simulink model "mpc2dof_lat_lon"  (R2022a)
settings: Solver=VariableStepAuto  StartTime=0.0  StopTime=5  RelTol=1e-3
PreLoadFcn:
  | preload
values from neighbouring files (symbols this model uses):
  aubr = [-8 -7.95 -7.9 -7.85 -7.8 -7.75 -7.7 -7.65 -7.6 -7.55 -7.5 -7.45 ... (261 elements, 1x261)]    [biaodingbiao.mat]
  tablebr = [-5.15763257253 -5.44224077841 -5.70856006024 -6.19075802128 -6.74229369367 -6.72484954572 -6.64837028644 -6.64755997194 -6.64688047281 -6.64617751235 -6.6454745519 -6.76173851825 ... (261261 elements, 1001x261)]    [biaodingbiao.mat]
  vubr = [0 0.05 0.1 0.15 0.2 0.25 0.3 0.35 0.4 0.45 0.5 0.55 ... (1001 elements, 1x1001)]    [biaodingbiao.mat]
libraries: slpidlib x3, Solver_SF x1
settings Model: Creator=化  LastModifiedBy=化

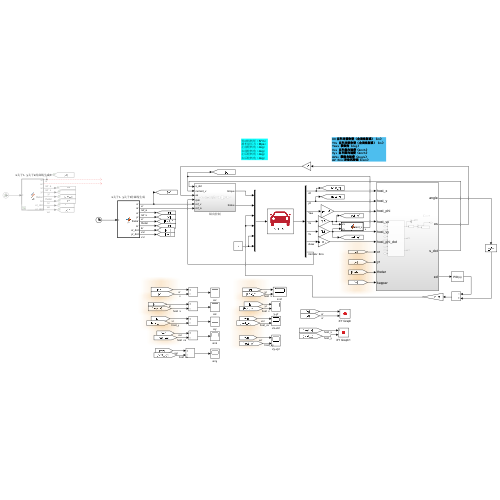
[thumbnail: Simulink's stored preview of the top-level diagram]
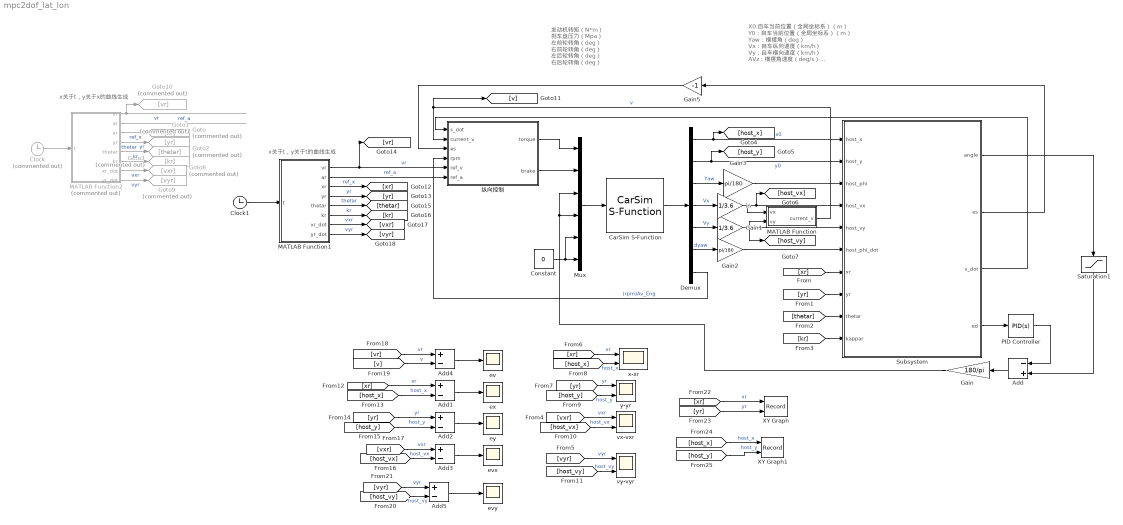
== system mpc2dof_lat_lon ==
  note: 发动机转矩（N*m）
      | 刹车盘压力（Mpa）
      | 左前轮转角（deg）
      | 右前轮转角（deg）
      | 左后轮转角（deg）
      | 右后轮转角（deg）
  note: X0:自车当前位置（全局坐标系）（m）
      | Y0：自车当前位置（全局坐标系）（m）
      | Yaw：横摆角（deg）
      | Vx：自车纵向速度（km/h）
      | Vy：自车横向速度（km/h）
      | AVz：横摆角速度（deg/s）
      | AV_Eng:发动机转速（rpm）
  note: x关于t，y关于x的曲线生成
  note: x关于t，y关于t的曲线生成
  Add : Sum  Inputs=-+
  Add{1..5} (5 alike) : Sum  Inputs=+-
  CarSim S-Function : Solver_SF/CarSim S-Function  Priority=1  SIMFILE=simfile.sim  Run_RTs=off  vs_state_ind=Run  StopMode_ind=Vehicle Model
  Clock : Clock  Commented=on
  Clock1 : Clock
  Constant : Constant  Value=0
  Demux : Demux  Outputs=7
  Gain : Gain  Gain=180/pi
  Gain1 : Gain  Gain=1/3.6
  Gain2 : Gain  Gain=pi/180
  Gain3 : Gain  Gain=pi/180
  Gain5 : Gain  Gain=-1
  Goto : Goto  Commented=on  GotoTag=xr
  Goto1 : Goto  Commented=on  GotoTag=yr
  Goto10 : Goto  Commented=on  GotoTag=vr
  Goto2 : Goto  Commented=on  GotoTag=thetar
  Goto3 : Goto  Commented=on  GotoTag=kr
  Goto8 : Goto  Commented=on  GotoTag=vxr
  Goto9 : Goto  Commented=on  GotoTag=vyr
  MATLAB Function : MATLAB Function  TreatAsAtomicUnit=on
  MATLAB Function1 : MATLAB Function  TreatAsAtomicUnit=on
  MATLAB Function2 : MATLAB Function  Commented=on  TreatAsAtomicUnit=on
  Mux : Mux  Inputs=6
  PID Controller : slpidlib/PID Controller  Controller=PID  Form=Parallel  TimeDomain=Continuous-time  UseExternalTs=off  SampleTime=-1  IntegratorMethod=Forward Euler  FilterMethod=Forward Euler  ControllerParametersSource=internal  P=0  I=3  UseKiTs=off  D=0  N=100  UseFilter=on  TunerSelectOption=Transfer Function Based (PID Tuner App)  InitialConditionSource=internal  InitialConditionForIntegrator=0  InitialConditionForFilter=0  DifferentiatorICPrevScaledInput=0  ExternalReset=none  TrackingMode=off  Kt=1  LimitOutput=off  SatLimitsSource=internal  UpperSaturationLimit=inf  LowerSaturationLimit=-inf  LinearizeAsGain=on  AntiWindupMode=none  Kb=1  POutMin=[]  POutMax=[]  IOutMin=[]  IOutMax=[]  DOutMin=[]  DOutMax=[]  NOutMin=[]  NOutMax=[]  SumOutMin=[]  SumOutMax=[]  SaturationOutMin=[]  SaturationOutMax=[]  PParamMin=[]  PParamMax=[]  IParamMin=[]  IParamMax=[]  DParamMin=[]  DParamMax=[]  NParamMin=[]  NParamMax=[]  KbParamMin=[]  KbParamMax=[]  KtParamMin=[]  KtParamMax=[]  KbOutMin=[]  KbOutMax=[]  KtOutMin=[]  KtOutMax=[]  IntegratorOutMin=[]  IntegratorOutMax=[]  FilterOutMin=[]  FilterOutMax=[]  SumI1OutMin=[]  SumI1OutMax=[]  SumI2OutMin=[]  SumI2OutMax=[]  SumI3OutMin=[]  SumI3OutMax=[]  SumI4OutMin=[]  SumI4OutMax=[]  SumDOutMin=[]  SumDOutMax=[]  DifferentiatorOutMin=[]  DifferentiatorOutMax=[]  FilterDiffOutCoefMin=[]  FilterDiffOutCoefMax=[]  ReciprocalOutMin=[]  ReciprocalOutMax=[]  SumDenOutMin=[]  SumDenOutMax=[]  SumNumOutMin=[]  SumNumOutMax=[]  DivideOutMin=[]  DivideOutMax=[]  UdiffTsProdOutMin=[]  UdiffTsProdOutMax=[]  NTsProdOutMin=[]  NTsProdOutMax=[]  UintegralTsProdOutMin=[]  UintegralTsProdOutMax=[]  UngainTsProdOutMin=[]  UngainTsProdOutMax=[]  IntegratorContinuousStateAttributes=''  IntegratorStateMustResolveToSignalObject=off  IntegratorRTWStateStorageClass=Auto  FilterContinuousStateAttributes=''  FilterStateMustResolveToSignalObject=off  FilterRTWStateStorageClass=Auto  ParallelPVariant=InternalParameters  IdealPVariant=Disabled  IVariant=InternalParameters  DVariant=InternalParameters  IntegratorVariant=Continuous  SatVariant=Disabled  AWVariant=Passthrough  PCopyVariant=Disabled  TRVariant=Disabled  FdbkBlocksVariant=Forward  IdealPFdbkVariant=Disabled  SatFdbkVariant=Disabled  DerivativeFilterVariant=ContFilter  NVariant=InternalParameters  NCopyVariant=Disabled  FilterICVariant=InternalICsFilter  IntegratorICVariant=InternalICs  ExternalResetVariant=Disabled  TRSumVariant=Passthrough  SumFdbkVariant=Disabled  SumVariant=Sum_PID  TsampFilterVariant=InternalTs  TsampNgainVariant=Passthrough  TsampIntegralVariant=Passthrough  ExternalSaturationOutDataTypeStr=Inherit: Same as second input  aMode=0
  Saturation1 : Saturate  UpperLimit=1  LowerLimit=-1
  Subsystem : Subsystem
  XY Graph : Record  FileSettingsInternal="{\"entries\":[{\"content\":{\"excelSettings\":{\"content\":{},\"type\":\"Streamout.ExcelSettings\"}},\"type\":\"Streamout.FileSettingStorage\",\"uuid\":\"0858db11-d2cd-44ce-b257-d2a84fc32b74\"}],\"packageUris\":[\"http://schema.mathworks.com/mf0/streamout_blocks/R2020a\"],\"version\":\"1.0\"}"  Layout=[1 1]  SignalsInternal="{\"entries\":[{\"content\":{\"signals\":[{\"content\":{\"blockPath\":[\"mpc2dof_lat_lon/XY Graph\"],\"channel\":[],\"dimensions\":[1],\"domain\":\"mpc2dof_lat_lon/XY Graph\",\"lineColor\":\"#a2142f\",\"plots\":[1],\"port\":1,\"sid\":[\"\"],\"signalID\":657,\"signalName\":\"xr\"},\"type\":\"RecordBlkView.Signal\",\"uuid\":\"f73990f6-9684-49e6-9729-589b4f1455ea\"},{\"content\":{\"blockPath\":[\"mpc2dof_lat_lon/XY Graph\"],\"channel\":[],\"dimensions\":[1],\"domain\":\"mpc2dof_lat_lon/XY Graph\",\"lineColor\":\"#139fff\",\"plots\":[1],\"port\":2,\"sid\":[\"\"],\"signalID\":661,\"signalName\":\"yr\"},\"type\":\"RecordBlkView.Signal\",\"uuid\":\"39c842ae-e1c5-41be-97e8-3fe2b4711ec7\"}]},\"type\":\"RecordBlkView.InputSignals\",\"uuid\":\"8e38f882-027b-4b6b-b800-43f1a68d75de\"}],\"packageUris\":[\"http://schema.mathworks.com/mf0/streamout_blocks/R2020a\"],\"version\":\"1.0\"}"  VisualizationBindings="{\"xyplotplugin\":{\"info\":[{\"series\":[{\"bindingParametersList\":[{\"parameter\":\"X-Axis\",\"signalID\":657,\"signalName\":\"xr\"},{\"parameter\":\"Y-Axis\",\"signalID\":661,\"signalName\":\"yr\"}],\"seriesID\":62107}],\"subplotID\":1}]}}"  CompatibilityTag=XY
  XY Graph1 : Record  FileSettingsInternal="{\"entries\":[{\"content\":{\"excelSettings\":{\"content\":{},\"type\":\"Streamout.ExcelSettings\"}},\"type\":\"Streamout.FileSettingStorage\",\"uuid\":\"ff16b887-db1a-418b-9102-38758cb726a0\"}],\"packageUris\":[\"http://schema.mathworks.com/mf0/streamout_blocks/R2020a\"],\"version\":\"1.0\"}"  Layout=[1 1]  SignalsInternal="{\"entries\":[{\"content\":{\"signals\":[{\"content\":{\"blockPath\":[\"mpc2dof_lat_lon/XY Graph1\"],\"channel\":[],\"dimensions\":[1],\"domain\":\"mpc2dof_lat_lon/XY Graph1\",\"lineColor\":\"#a2142f\",\"plots\":[1],\"port\":1,\"sid\":[\"\"],\"signalID\":665,\"signalName\":\"host_x\"},\"type\":\"RecordBlkView.Signal\",\"uuid\":\"320865bc-cbe4-4e56-b7b5-0f52d94d4ba8\"},{\"content\":{\"blockPath\":[\"mpc2dof_lat_lon/XY Graph1\"],\"channel\":[],\"dimensions\":[1],\"domain\":\"mpc2dof_lat_lon/XY Graph1\",\"lineColor\":\"#139fff\",\"plots\":[1],\"port\":2,\"sid\":[\"\"],\"signalID\":669,\"signalName\":\"host_y\"},\"type\":\"RecordBlkView.Signal\",\"uuid\":\"5f5de268-9097-4b48-9093-019a8f4207d0\"}]},\"type\":\"RecordBlkView.InputSignals\",\"uuid\":\"43d80a1c-d21a-445c-991d-4928644d10b0\"}],\"packageUris\":[\"http://schema.mathworks.com/mf0/streamout_blocks/R2020a\"],\"version\":\"1.0\"}"  VisualizationBindings="{\"xyplotplugin\":{\"info\":[{\"series\":[{\"bindingParametersList\":[{\"parameter\":\"X-Axis\",\"signalID\":665,\"signalName\":\"host_x\"},{\"parameter\":\"Y-Axis\",\"signalID\":669,\"signalName\":\"host_y\"}],\"seriesID\":16940}],\"subplotID\":1}]}}"  CompatibilityTag=XY
  ev : Scope
  evx : Scope
  evy : Scope
  ex : Scope
  ey : Scope
  in : Gain  Gain=1/3.6
  vx-vxr : Scope  NumInputPorts=2
  vy-vyr : Scope  NumInputPorts=2
  x-xr : Scope  NumInputPorts=2
  y-yr : Scope  NumInputPorts=2
  纵向控制 : Subsystem
  wires:
  Demux/5 -> Gain1/1  "Vy"
  Demux/6 -> Gain2/1  "dyaw"
  Demux/4 -> in/1  "Vx"
  Demux/3 -> Gain3/1  "Yaw"
  CarSim S-Function/1 -> Demux/1
  纵向控制/2(brake) -> Mux/2
  纵向控制/1(torque) -> Mux/1
  Constant/1 -> Mux/5, Mux/6
  in/1 -> [host_vx], Subsystem/4(host_vx), MATLAB Function/1(vx)
  Gain1/1 -> [host_vy], Subsystem/5(host_vy), MATLAB Function/2(vy)
  MATLAB Function/1(current_v) -> [v], 纵向控制/2(current_v)  "v"
  Demux/1 -> [host_x], Subsystem/1(host_x)  "x0"
  Demux/2 -> [host_y], Subsystem/2(host_y)  "y0"
  Gain3/1 -> Subsystem/3(host_phi)
  Gain2/1 -> Subsystem/6(host_phi_dot)
  Demux/7 -> 纵向控制/4(rpm)  "(rpm)Av_Eng"
  Subsystem/2(es) -> Gain5/1
  Subsystem/3(s_dot) -> 纵向控制/1(s_dot)
  [xr] -> Subsystem/7(xr)
  [yr] -> Subsystem/8(yr)
  [kr] -> Subsystem/10(kappar)
  [thetar] -> Subsystem/9(thetar)
  Gain5/1 -> 纵向控制/3(es)
  [xr] -> x-xr/1  "xr"
  [host_x] -> x-xr/2  "host_x"
  [yr] -> y-yr/1  "yr"
  [host_y] -> y-yr/2  "host_y"
  [host_vx] -> vx-vxr/2  "host_vx"
  [vxr] -> vx-vxr/1  "vxr"
  [vyr] -> vy-vyr/1  "vyr"
  [host_vy] -> vy-vyr/2  "host_vy"
  Subsystem/1(angle) -> Saturation1/1
  Saturation1/1 -> Add/2
  Subsystem/4(ed) -> PID Controller/1
  PID Controller/1 -> Add/1
  Add/1 -> Gain/1
  Gain/1 -> Mux/3, Mux/4
  [xr] -> Add1/1  "xr"
  [host_x] -> Add1/2  "host_x"
  Add1/1 -> ex/1
  [yr] -> Add2/1  "yr"
  [host_y] -> Add2/2  "host_y"
  Add2/1 -> ey/1
  [vxr] -> Add3/1  "vxr"
  [host_vx] -> Add3/2  "host_vx"
  Add3/1 -> evx/1
  [vr] -> Add4/1  "vr"
  [v] -> Add4/2  "v"
  Add4/1 -> ev/1
  Mux/1 -> CarSim S-Function/1
  MATLAB Function1/8(yr_dot) -> [vyr]  "vyr"
  MATLAB Function1/3(xr) -> [xr]  "ref_x"
  MATLAB Function1/4(yr) -> [yr]  "yr"
  MATLAB Function1/5(thetar) -> [thetar]  "thetar"
  MATLAB Function1/6(kr) -> [kr]  "kr"
  MATLAB Function1/7(xr_dot) -> [vxr]  "vxr"
  MATLAB Function2/2(ar) -> ?  "ref_a"
  MATLAB Function2/6(kr) -> Goto3/1  "kr"
  Clock/1 -> MATLAB Function2/1(t)
  MATLAB Function2/7(xr_dot) -> Goto8/1  "vxr"
  MATLAB Function2/8(yr_dot) -> Goto9/1  "vyr"
  MATLAB Function2/3(xr) -> Goto/1  "ref_x"
  MATLAB Function2/1(vr) -> Goto10/1  "vr"
  MATLAB Function2/5(thetar) -> Goto2/1  "thetar"
  MATLAB Function2/4(yr) -> Goto1/1  "yr"
  MATLAB Function1/1(vr) -> [vr], 纵向控制/5(ref_v)  "vr"
  MATLAB Function1/2(ar) -> 纵向控制/6(ref_a)  "ref_a"
  Clock1/1 -> MATLAB Function1/1(t)
  [host_vy] -> Add5/2  "host_vy"
  [vyr] -> Add5/1  "vyr"
  Add5/1 -> evy/1
  [xr] -> XY Graph/1  "xr"
  [yr] -> XY Graph/2  "yr"
  [host_x] -> XY Graph1/1  "host_x"
  [host_y] -> XY Graph1/2  "host_y"

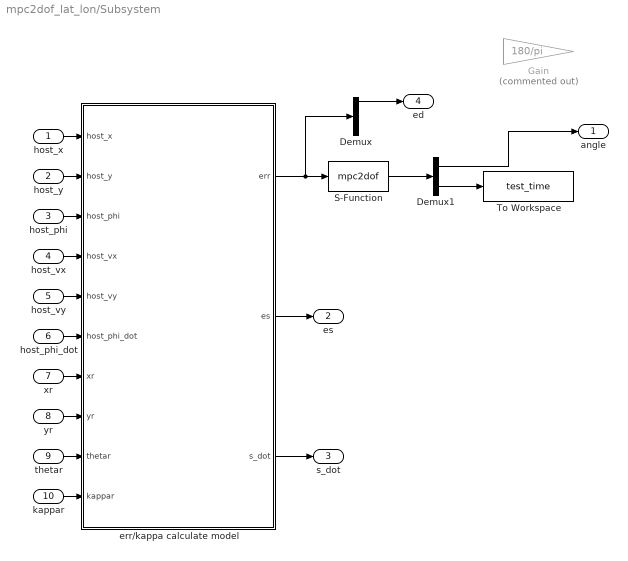
== system mpc2dof_lat_lon/Subsystem ==
  host_x : Inport
  host_y : Inport  Port=2
  host_phi : Inport  Port=3
  host_vx : Inport  Port=4
  host_vy : Inport  Port=5
  host_phi_dot : Inport  Port=6
  xr : Inport  Port=7
  yr : Inport  Port=8
  thetar : Inport  Port=9
  kappar : Inport  Port=10
  Demux : Demux
  Demux1 : Demux  Outputs=2
  Gain : Gain  Commented=on  Gain=180/pi
  S-Function : S-Function  FunctionName=mpc2dof  SFunctionDeploymentMode=off  EnableBusSupport=off
  To Workspace : ToWorkspace  VariableName=test_time  SaveFormat=Timeseries  SampleTime=-1
  err/kappa calculate model : MATLAB Function  TreatAsAtomicUnit=on
  angle : Outport
  es : Outport  Port=2
  s_dot : Outport  Port=3
  ed : Outport  Port=4
  wires:
  host_x/1 -> err/kappa calculate model/1(host_x)
  S-Function/1 -> Demux1/1
  Demux1/1 -> angle/1
  host_y/1 -> err/kappa calculate model/2(host_y)
  Demux1/2 -> To Workspace/1
  host_vx/1 -> err/kappa calculate model/4(host_vx)
  host_vy/1 -> err/kappa calculate model/5(host_vy)
  host_phi/1 -> err/kappa calculate model/3(host_phi)
  thetar/1 -> err/kappa calculate model/9(thetar)
  host_phi_dot/1 -> err/kappa calculate model/6(host_phi_dot)
  yr/1 -> err/kappa calculate model/8(yr)
  kappar/1 -> err/kappa calculate model/10(kappar)
  xr/1 -> err/kappa calculate model/7(xr)
  err/kappa calculate model/2(es) -> es/1
  err/kappa calculate model/3(s_dot) -> s_dot/1
  Demux/1 -> ed/1
  err/kappa calculate model/1(err) -> Demux/1, S-Function/1

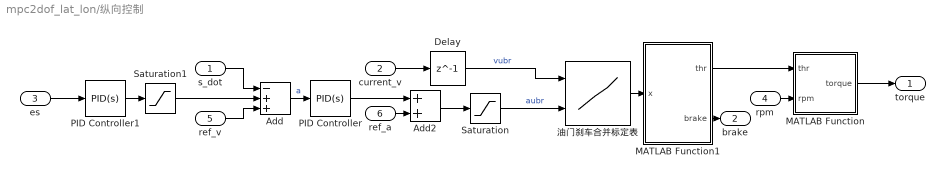
== system mpc2dof_lat_lon/纵向控制 ==
  s_dot : Inport
  current_v : Inport  Port=2
  es : Inport  Port=3
  rpm : Inport  Port=4
  ref_v : Inport  Port=5
  ref_a : Inport  Port=6
  Add : Sum  Inputs=-++
  Add2 : Sum
  Delay : Delay  DelayLength=1
  MATLAB Function : MATLAB Function  TreatAsAtomicUnit=on
  MATLAB Function1 : MATLAB Function  TreatAsAtomicUnit=on
  PID Controller : slpidlib/PID Controller  Controller=PID  Form=Parallel  TimeDomain=Continuous-time  UseExternalTs=off  SampleTime=-1  IntegratorMethod=Forward Euler  FilterMethod=Forward Euler  ControllerParametersSource=internal  P=1  I=0  UseKiTs=off  D=0.1  N=100  UseFilter=on  TunerSelectOption=Transfer Function Based (PID Tuner App)  InitialConditionSource=internal  InitialConditionForIntegrator=0  InitialConditionForFilter=0  DifferentiatorICPrevScaledInput=0  ExternalReset=none  TrackingMode=off  Kt=1  LimitOutput=off  SatLimitsSource=internal  UpperSaturationLimit=inf  LowerSaturationLimit=-inf  LinearizeAsGain=on  AntiWindupMode=none  Kb=1  POutMin=[]  POutMax=[]  IOutMin=[]  IOutMax=[]  DOutMin=[]  DOutMax=[]  NOutMin=[]  NOutMax=[]  SumOutMin=[]  SumOutMax=[]  SaturationOutMin=[]  SaturationOutMax=[]  PParamMin=[]  PParamMax=[]  IParamMin=[]  IParamMax=[]  DParamMin=[]  DParamMax=[]  NParamMin=[]  NParamMax=[]  KbParamMin=[]  KbParamMax=[]  KtParamMin=[]  KtParamMax=[]  KbOutMin=[]  KbOutMax=[]  KtOutMin=[]  KtOutMax=[]  IntegratorOutMin=[]  IntegratorOutMax=[]  FilterOutMin=[]  FilterOutMax=[]  SumI1OutMin=[]  SumI1OutMax=[]  SumI2OutMin=[]  SumI2OutMax=[]  SumI3OutMin=[]  SumI3OutMax=[]  SumI4OutMin=[]  SumI4OutMax=[]  SumDOutMin=[]  SumDOutMax=[]  DifferentiatorOutMin=[]  DifferentiatorOutMax=[]  FilterDiffOutCoefMin=[]  FilterDiffOutCoefMax=[]  ReciprocalOutMin=[]  ReciprocalOutMax=[]  SumDenOutMin=[]  SumDenOutMax=[]  SumNumOutMin=[]  SumNumOutMax=[]  DivideOutMin=[]  DivideOutMax=[]  UdiffTsProdOutMin=[]  UdiffTsProdOutMax=[]  NTsProdOutMin=[]  NTsProdOutMax=[]  UintegralTsProdOutMin=[]  UintegralTsProdOutMax=[]  UngainTsProdOutMin=[]  UngainTsProdOutMax=[]  IntegratorContinuousStateAttributes=''  IntegratorStateMustResolveToSignalObject=off  IntegratorRTWStateStorageClass=Auto  FilterContinuousStateAttributes=''  FilterStateMustResolveToSignalObject=off  FilterRTWStateStorageClass=Auto  ParallelPVariant=InternalParameters  IdealPVariant=Disabled  IVariant=InternalParameters  DVariant=InternalParameters  IntegratorVariant=Continuous  SatVariant=Disabled  AWVariant=Passthrough  PCopyVariant=Disabled  TRVariant=Disabled  FdbkBlocksVariant=Forward  IdealPFdbkVariant=Disabled  SatFdbkVariant=Disabled  DerivativeFilterVariant=ContFilter  NVariant=InternalParameters  NCopyVariant=Disabled  FilterICVariant=InternalICsFilter  IntegratorICVariant=InternalICs  ExternalResetVariant=Disabled  TRSumVariant=Passthrough  SumFdbkVariant=Disabled  SumVariant=Sum_PID  TsampFilterVariant=InternalTs  TsampNgainVariant=Passthrough  TsampIntegralVariant=Passthrough  ExternalSaturationOutDataTypeStr=Inherit: Same as second input  aMode=0
  PID Controller1 : slpidlib/PID Controller  Controller=PID  Form=Parallel  TimeDomain=Continuous-time  UseExternalTs=off  SampleTime=-1  IntegratorMethod=Forward Euler  FilterMethod=Forward Euler  ControllerParametersSource=internal  P=3  I=0  UseKiTs=off  D=0.1  N=30  UseFilter=on  TunerSelectOption=Transfer Function Based (PID Tuner App)  InitialConditionSource=internal  InitialConditionForIntegrator=0  InitialConditionForFilter=0  DifferentiatorICPrevScaledInput=0  ExternalReset=none  TrackingMode=off  Kt=1  LimitOutput=off  SatLimitsSource=internal  UpperSaturationLimit=inf  LowerSaturationLimit=-inf  LinearizeAsGain=on  AntiWindupMode=none  Kb=1  POutMin=[]  POutMax=[]  IOutMin=[]  IOutMax=[]  DOutMin=[]  DOutMax=[]  NOutMin=[]  NOutMax=[]  SumOutMin=[]  SumOutMax=[]  SaturationOutMin=[]  SaturationOutMax=[]  PParamMin=[]  PParamMax=[]  IParamMin=[]  IParamMax=[]  DParamMin=[]  DParamMax=[]  NParamMin=[]  NParamMax=[]  KbParamMin=[]  KbParamMax=[]  KtParamMin=[]  KtParamMax=[]  KbOutMin=[]  KbOutMax=[]  KtOutMin=[]  KtOutMax=[]  IntegratorOutMin=[]  IntegratorOutMax=[]  FilterOutMin=[]  FilterOutMax=[]  SumI1OutMin=[]  SumI1OutMax=[]  SumI2OutMin=[]  SumI2OutMax=[]  SumI3OutMin=[]  SumI3OutMax=[]  SumI4OutMin=[]  SumI4OutMax=[]  SumDOutMin=[]  SumDOutMax=[]  DifferentiatorOutMin=[]  DifferentiatorOutMax=[]  FilterDiffOutCoefMin=[]  FilterDiffOutCoefMax=[]  ReciprocalOutMin=[]  ReciprocalOutMax=[]  SumDenOutMin=[]  SumDenOutMax=[]  SumNumOutMin=[]  SumNumOutMax=[]  DivideOutMin=[]  DivideOutMax=[]  UdiffTsProdOutMin=[]  UdiffTsProdOutMax=[]  NTsProdOutMin=[]  NTsProdOutMax=[]  UintegralTsProdOutMin=[]  UintegralTsProdOutMax=[]  UngainTsProdOutMin=[]  UngainTsProdOutMax=[]  IntegratorContinuousStateAttributes=''  IntegratorStateMustResolveToSignalObject=off  IntegratorRTWStateStorageClass=Auto  FilterContinuousStateAttributes=''  FilterStateMustResolveToSignalObject=off  FilterRTWStateStorageClass=Auto  ParallelPVariant=InternalParameters  IdealPVariant=Disabled  IVariant=InternalParameters  DVariant=InternalParameters  IntegratorVariant=Continuous  SatVariant=Disabled  AWVariant=Passthrough  PCopyVariant=Disabled  TRVariant=Disabled  FdbkBlocksVariant=Forward  IdealPFdbkVariant=Disabled  SatFdbkVariant=Disabled  DerivativeFilterVariant=ContFilter  NVariant=InternalParameters  NCopyVariant=Disabled  FilterICVariant=InternalICsFilter  IntegratorICVariant=InternalICs  ExternalResetVariant=Disabled  TRSumVariant=Passthrough  SumFdbkVariant=Disabled  SumVariant=Sum_PID  TsampFilterVariant=InternalTs  TsampNgainVariant=Passthrough  TsampIntegralVariant=Passthrough  ExternalSaturationOutDataTypeStr=Inherit: Same as second input  aMode=0
  Saturation : Saturate  UpperLimit=5  LowerLimit=-8
  Saturation1 : Saturate  UpperLimit=10  LowerLimit=-10
  油门刹车合并标定表 : Lookup_n-D  BreakpointsForDimension1=vubr  BreakpointsForDimension2=aubr  Table=tablebr  InternalRulePriority=Speed  RndMeth=Simplest
      settings: InputPortMap=u0,u1
  torque : Outport
  brake : Outport  Port=2
  wires:
  Delay/1 -> 油门刹车合并标定表/1  "vubr"
  Add/1 -> PID Controller/1  "a"
  ref_v/1 -> Add/3
  ref_a/1 -> Add2/2
  油门刹车合并标定表/1 -> MATLAB Function1/1(x)
  PID Controller1/1 -> Saturation1/1
  PID Controller/1 -> Add2/1
  Add2/1 -> Saturation/1
  Saturation1/1 -> Add/2
  Saturation/1 -> 油门刹车合并标定表/2  "aubr"
  MATLAB Function1/1(thr) -> MATLAB Function/1(thr)
  s_dot/1 -> Add/1
  current_v/1 -> Delay/1
  es/1 -> PID Controller1/1
  rpm/1 -> MATLAB Function/2(rpm)
  MATLAB Function/1(torque) -> torque/1
  MATLAB Function1/2(brake) -> brake/1

== matlab function mpc2dof_lat_lon/纵向控制/MATLAB Function1 ==
  data: x input; thr output; brake output
function [thr,brake] = fcn(x)
% 正数代表油门，负数代表刹车
% 不允许同时踩油门和刹车
    if x>=0
        thr=x;
        brake=0;
    else
        brake=-x;
        thr=0;
    end
end

== matlab function mpc2dof_lat_lon/纵向控制/MATLAB Function ==
  data: thr input; torque output; rpm input
function torque  = fcn(thr,rpm)
Tmax=380*thr;
    if(rpm<=4523)
        torque=Tmax;
    else
        torque=Tmax*4523/rpm;
    end
end

== matlab function mpc2dof_lat_lon/MATLAB Function2 ==
  data: vr output; ar output; t input; xr output; yr output; thetar output; kr output; xr_dot output; yr_dot output
function [vr,ar,xr,yr,thetar,kr,xr_dot,yr_dot] = fcn(t)
    dx=100;
    %dy=3.75;
    dy=10;
    T=20;
    %x，y起点终点位置
    xstart=[0,0,0];
    xend=[dx,0,0];
    ystart=[0,0,0];
    yend=[dy,0,0];
    %系数初始化
    a=zeros(1,6);
    b=zeros(1,6);
    % 五次多项式A系数矩阵
    a(1)=xstart(1);
    a(2)=xstart(2);
    a(3)=xstart(3)/2;
    %求解剩下三个系数
    A1=[T^3 , T^4 , T^5;
        3*T^2,4*T^3,5*T^4;
        6*T,12*T^2,20*T^3];
    B1=[xend(1)-a(1)-a(2)*T-a(3)*T^2;
        xend(2)-a(2)-2*a(3)*T;
        xend(3)-2*a(3)];
    xs=A1\B1;
    a(4)=xs(1);
    a(5)=xs(2);
    a(6)=xs(3);
    % 五次多项式B系数矩阵求解
    b(1)=ystart(1);
    b(2)=ystart(2);
    b(3)=ystart(3)/2;
    %求解剩下三个系数
    A2=[dx^3 , dx^4 , dx^5;
        3*dx^2,4*dx^3,5*dx^4;
        6*dx,12*dx^2,20*dx^3];
    B2=[yend(1)-b(1)-b(2)*dx-b(3)*dx^2;
        yend(2)-b(2)-2*b(3)*dx;
        yend(3)-2*b(3)];
    ys=A2\B2;
    b(4)=ys(1);
    b(5)=ys(2);
    b(6)=ys(3);

    %xr,yr（位置参考值）
    xr=a(1)+a(2)*t+a(3)*t^2+a(4)*t^3+a(5)*t^4+a(6)*t^5;
    yr=b(1)+b(2)*xr+b(3)*xr^2+b(4)*xr^3+b(5)*xr^4+b(6)*xr^5;
    %xr_dot（vx参考值） , yr_dx
    xr_dot=a(2)+2*a(3)*t+3*a(4)*t^2+4*a(5)*t^3+5*a(6)*t^4;
    yr_dx=b(2)+2*b(3)*xr+3*b(4)*xr^2+4*b(5)*xr^3+5*b(6)*xr^4;
    %yr_dot（vy参考值）
    yr_dot=yr_dx*xr_dot;
    %thetar（航向角参考值）
    thetar=atan(yr_dx);
    %xr_dot_dot（ax参考值）
    xr_dot2=2*a(3)+6*a(4)*t+12*a(5)*t^2+20*a(6)*t^3;
    %yr_dx_dx
    yr_dx2=2*b(3)+6*b(4)*xr+12*b(5)*xr^2+20*b(6)*xr^3;
    %yr_dot_dot（ay参考值）
    yr_dot2=yr_dx2*xr_dot^2+yr_dx*xr_dot2;
    %kr(曲率参考值)
    kr=yr_dx2/((1+yr_dx^2)^1.5);
    %速度参考值
    vr=sqrt(xr_dot^2+yr_dot^2);
    %如果加速度大于0
    if xr_dot2>=0
        ar=sqrt(xr_dot2^2+yr_dot2^2);
    else
        ar=-sqrt(xr_dot2^2+yr_dot2^2);
    end

== matlab function mpc2dof_lat_lon/MATLAB Function ==
  data: vx input; current_v output; vy input
function current_v = fcn(vx,vy)
current_v=sqrt(vx^2+vy^2);

== matlab function mpc2dof_lat_lon/MATLAB Function1 ==
  data: t input; vr output; ar output; xr output; yr output; thetar output; kr output; xr_dot output; yr_dot output
function [vr,ar,xr,yr,thetar,kr,xr_dot,yr_dot] = fcn(t)
    tau=5;
    w=3.75;
    vx=20;  %m/s
    %系数初始化
    
    xr=vx*t;
    yr=10*w*t^3/tau^3 - 15*w*t^4/tau^4 + 6*w*t^5/tau^5;

    xr_dot=vx;
    xr_dot_dot=0;

    yr_dot=30*w*t^2/tau^3 - 60*w*t^3/tau^4 + 30*w*t^4/tau^5;
    yr_dot_dot=60*w*t/tau^3 - 180*w*t^2/tau^4 + 120*w*t^3/tau^5;

    thetar=yr_dot/xr_dot;
    kr=abs(xr_dot*yr_dot_dot-yr_dot*xr_dot_dot)/((xr_dot^2+yr_dot^2)^1.5);

    vr=sqrt(xr_dot^2 + yr_dot^2);
    if xr_dot_dot>=0
        ar=sqrt(xr_dot_dot^2+yr_dot_dot^2);
    else
        ar=-sqrt(xr_dot_dot^2+yr_dot_dot^2);
    end

== matlab function mpc2dof_lat_lon/Subsystem/err//kappa calculate model ==
  data: host_x input; err output; host_y input; host_phi input; host_vx input; host_vy input; host_phi_dot input; xr input; yr input; thetar input; kappar input; es output; s_dot output
function [err,es,s_dot]  = fcn(host_x,host_y,host_phi,host_vx,host_vy,host_phi_dot,xr,yr,thetar,kappar)
%%%[err,kappa,es,s_dot]     
%计算投影点到匹配点之间的err kappa es s_dot

    %匹配点的法向量 切向量
    tor=[cos(thetar);sin(thetar)];
    nor=[-sin(thetar);cos(thetar)];
    %自车到匹配点的向量距离
    d_err=[host_x-xr;host_y-yr];
    %自车到匹配点的横向距离
    ed=nor'*d_err;
    %自车到匹配点的纵向距离
    es=tor'*d_err;
    %apollo中对投影点的航向角的定义
    %projection_point_thetar=thetar(dmin);

    %老王对投影点的航向角的定义
    projection_point_thetar=thetar+kappar*es;
    %切向速度
    ed_dot=host_vy*cos(host_phi-projection_point_thetar)+host_vx*sin(host_phi-projection_point_thetar);
    %自车到投影点的横摆角差值
    ephi=sin(host_phi-projection_point_thetar);
    %求出s_dot
    ss_dot=host_vx*cos(host_phi-projection_point_thetar)-host_vy*sin(host_phi-projection_point_thetar);
    s_dot=ss_dot/(1-kappar*ed);
    %求出ephi_dot
    ephi_dot=host_phi_dot-kappar*s_dot;
    %kappa=kappar;
    err=[ed;ed_dot;ephi;ephi_dot];

end
